simulink model "Plant_d_Bench"  (R2024b)
settings: Solver=FixedStepDiscrete  StartTime=0.0  StopTime=10.0  FixedStep=0.01  RelTol=1e-3
model workspace (MATLAB code in the model file):
  | AllParams;
settings Model: Creator=marijn  LastModifiedBy=marijn

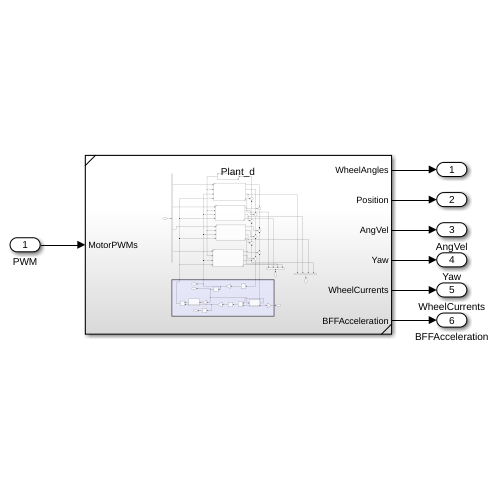
[thumbnail: Simulink's stored preview of the top-level diagram]
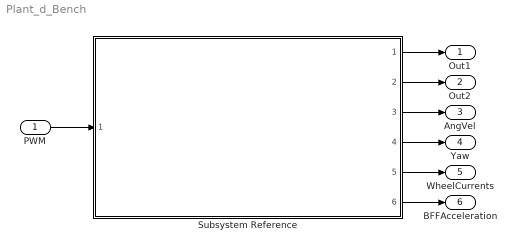
== system Plant_d_Bench ==
  PWM : Inport  PortDimensions=4
  Subsystem Reference : Subsystem  ReferencedSubsystem=Plant_d
  Out1 : Outport
  Out2 : Outport  Port=2
  AngVel : Outport  Port=3
  Yaw : Outport  Port=4
  WheelCurrents : Outport  Port=5
  BFFAcceleration : Outport  Port=6
  wires:
  PWM/1 -> Subsystem Reference/1
  Subsystem Reference/1 -> Out1/1
  Subsystem Reference/2 -> Out2/1
  Subsystem Reference/3 -> AngVel/1
  Subsystem Reference/4 -> Yaw/1
  Subsystem Reference/5 -> WheelCurrents/1
  Subsystem Reference/6 -> BFFAcceleration/1
